simulink model "painel"  (R2017b)
settings: Solver=VariableStepAuto  StartTime=0.0  StopTime=200  RelTol=1e-3
libraries: simulink x2
settings Model: Creator=vbob  LastModifiedBy=vbob

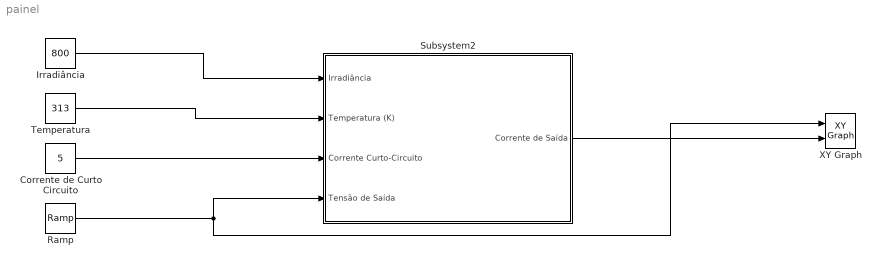
== system painel ==
  Corrente de Curto Circuito : Constant  Value=5
  Irradiância : Constant  Value=800
  Ramp : simulink/Sources/Ramp  slope=0.01  start=0  X0=0
  Subsystem2 : Subsystem
  Temperatura : Constant  Value=313
  XY Graph : simulink/Sinks/XY Graph  xmin=0  xmax=2  ymin=0  ymax=5  st=-1
  wires:
  Irradiância/1 -> Subsystem2/1(Irradiância)
  Temperatura/1 -> Subsystem2/2(Temperatura (K))
  Corrente de Curto Circuito/1 -> Subsystem2/3(Corrente Curto-Circuito)
  Ramp/1 -> XY Graph/1, Subsystem2/4(Tensão de Saída)
  Subsystem2/1(Corrente de Saída) -> XY Graph/2

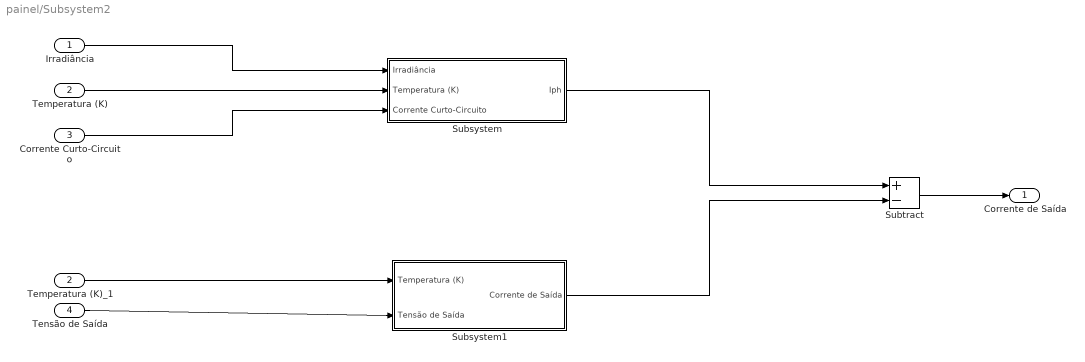
== system painel/Subsystem2 ==
  Irradiância : Inport
  Temperatura (K) : Inport  Port=2
  Corrente Curto-Circuito : Inport  Port=3
  Tensão de Saída : Inport  Port=4
  Subsystem : Subsystem  mask{R=800, T=313, ICC=5}
      mask prompts: R "Irradiância"; T "Temperatura"; ICC "Corrento Curto-Circuito"
  Subsystem1 : Subsystem  mask{V=0}
      mask prompts: V "Tensão de Saída"
  Subtract : Sum  Inputs=+-
  Temperatura (K)_1 : InportShadow  Port=2
  Corrente de Saída : Outport
  wires:
  Irradiância/1 -> Subsystem/1(Irradiância)
  Subsystem/1(Iph) -> Subtract/1
  Temperatura (K)/1 -> Subsystem/2(Temperatura (K))
  Corrente Curto-Circuito/1 -> Subsystem/3(Corrente Curto-Circuito)
  Tensão de Saída/1 -> Subsystem1/2(Tensão de Saída)
  Temperatura (K)_1/1 -> Subsystem1/1(Temperatura (K))
  Subsystem1/1(Corrente de Saída) -> Subtract/2
  Subtract/1 -> Corrente de Saída/1

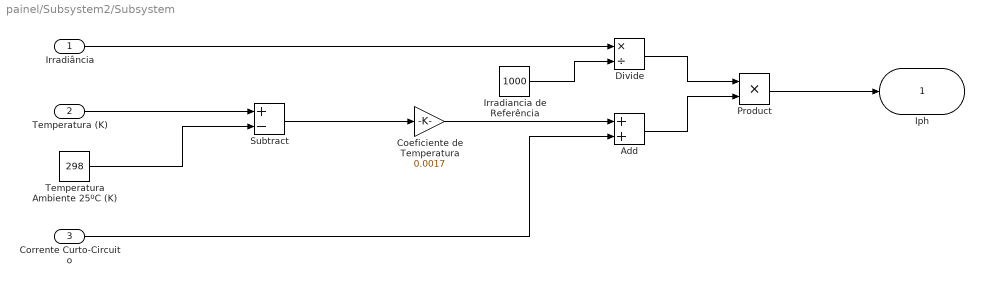
== system painel/Subsystem2/Subsystem ==
  Irradiância : Inport
  Temperatura (K) : Inport  Port=2
  Corrente Curto-Circuito : Inport  Port=3
  Add : Sum
  Coeficiente de Temperatura : Gain  Gain=0.0017
  Divide : Product  Inputs=*/
  "Irradiancia de Referência " : Constant  Value=1000
  Product : Product
  Subtract : Sum  Inputs=+-
  Temperatura Ambiente 25ºC (K) : Constant  Value=298
  Iph : Outport
  wires:
  Divide/1 -> Product/1
  Add/1 -> Product/2
  Product/1 -> Iph/1
  Corrente Curto-Circuito/1 -> Add/2
  Coeficiente de Temperatura/1 -> Add/1
  Temperatura (K)/1 -> Subtract/1
  Irradiância/1 -> Divide/1
  Subtract/1 -> Coeficiente de Temperatura/1
  Temperatura Ambiente 25ºC (K)/1 -> Subtract/2
  "Irradiancia de Referência "/1 -> Divide/2

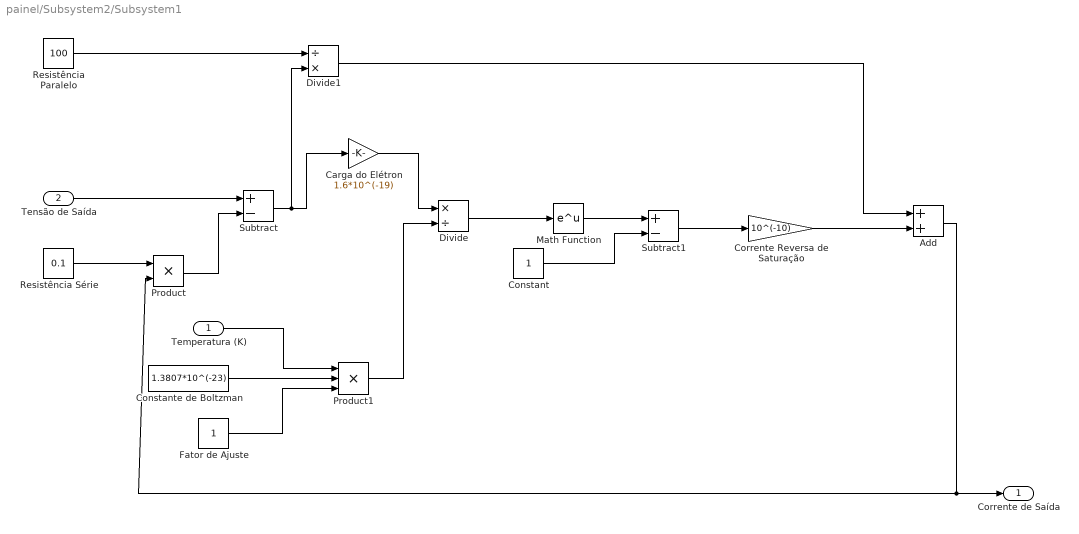
== system painel/Subsystem2/Subsystem1 ==
  Temperatura (K) : Inport
  Tensão de Saída : Inport  Port=2
  Add : Sum
  Carga do Elétron : Gain  Gain=1.6*10^(-19)
  Constant : Constant
  Constante de Boltzman : Constant  Value=1.3807*10^(-23)
  Corrente Reversa de Saturação : Gain  Gain=10^(-10)
  Divide : Product  Inputs=*/
  Divide1 : Product  Inputs=/*
  "Fator de Ajuste " : Constant
  Math Function : Math  SaturateOnIntegerOverflow=on
  Product : Product
  Product1 : Product  Inputs=3
  Resistência Paralelo : Constant  Value=100
  Resistência Série : Constant  Value=0.1
  Subtract : Sum  Inputs=+-
  Subtract1 : Sum  Inputs=+-
  Corrente de Saída : Outport
  wires:
  Subtract1/1 -> Corrente Reversa de Saturação/1
  Divide1/1 -> Add/1
  Divide/1 -> Math Function/1
  "Fator de Ajuste "/1 -> Product1/3
  Add/1 -> Corrente de Saída/1, Product/2
  Corrente Reversa de Saturação/1 -> Add/2
  Constant/1 -> Subtract1/2
  Carga do Elétron/1 -> Divide/1
  Temperatura (K)/1 -> Product1/1
  Constante de Boltzman/1 -> Product1/2
  Tensão de Saída/1 -> Subtract/1
  Math Function/1 -> Subtract1/1
  Resistência Série/1 -> Product/1
  Product1/1 -> Divide/2
  Resistência Paralelo/1 -> Divide1/1
  Product/1 -> Subtract/2
  Subtract/1 -> Divide1/2, Carga do Elétron/1
